simulink model "EEG_2022_040_Simulink_ex2"  (R2024a)
settings: Solver=VariableStepAuto  StartTime=0.0  StopTime=10.0  RelTol=1e-3
settings Model: Creator=User  LastModifiedBy=User

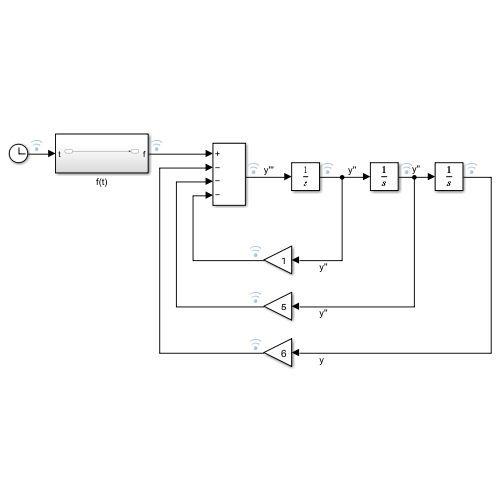
[thumbnail: Simulink's stored preview of the top-level diagram]
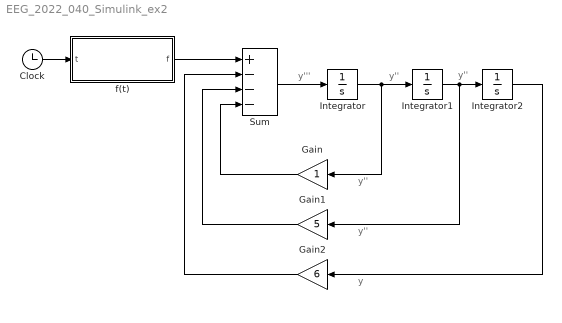
== system EEG_2022_040_Simulink_ex2 ==
  note: y'''
  note: y''
  note: y
  note: y''
  note: y''
  note: y''
  Clock : Clock
  Gain : Gain
  Gain1 : Gain  Gain=5
  Gain2 : Gain  Gain=6
  Integrator : Integrator
  Integrator1 : Integrator
  Integrator2 : Integrator
  Sum : Sum  Inputs=+---
  f(t) : Subsystem
  wires:
  Clock/1 -> f(t)/1(t)
  f(t)/1(f) -> Sum/1
  Sum/1 -> Integrator/1
  Integrator/1 -> Gain/1, Integrator1/1
  Integrator1/1 -> Integrator2/1, Gain1/1
  Integrator2/1 -> Gain2/1
  Gain/1 -> Sum/4
  Gain1/1 -> Sum/3
  Gain2/1 -> Sum/2

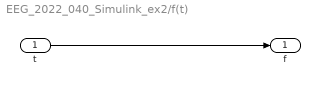
== system EEG_2022_040_Simulink_ex2/f(t) ==
  t : Inport
  f : Outport
  wires:
  t/1 -> f/1
